simulink model "Model_6DOF_B3"  (R2020b)
settings: Solver=FixedStepAuto  StartTime=0.0  StopTime=120  FixedStep=0.05  RelTol=1e-3
values from neighbouring files (symbols this model uses):
  Ba_0 = [0 0 0 0 0 0]    [ctrl_mode_param.m]
  Bb = 4418825.3321    [load_data.m]
  Bv_0 = [tgt_speed 0 0 0 0 0]    [ctrl_mode_param.m]
  Bx_0 = [0 0 tgt_depth 0 0 0]    [ctrl_mode_param.m]
  Ixx = 5.23e7    (= 52300000)    [load_data.m]
  Ixy = 0    [load_data.m]
  Ixz = 0    [load_data.m]
  Iyy = 1.375e9    (= 1375000000)    [load_data.m]
  Iyz = 0    [load_data.m]
  Izz = 1.367e9    (= 1367000000)    [load_data.m]
  Mb = 4418825.3321    [load_data.m]
  Xb = 0    [load_data.m]
  Xg = 0    [load_data.m]
  Yb = 0    [load_data.m]
  Yg = 0    [load_data.m]
  Zb = 0.4406    [load_data.m]
  Zg = 0    [load_data.m]
undefined symbols (not defined in the file or in its folder): dA_BP1, dA_BP2, dA_Hull, dA_PH, dA_Sail, dA_SProot, dA_X1a, dA_X1b, dA_X2a, dA_X2b, dA_X3a, dA_X3b, dA_X4a, dA_X4b, its, n_BP1, n_BP2, n_Hull, n_PH, n_Sail, n_SProot, n_X1a, n_X1b, n_X2a, n_X2b, n_X3a, n_X3b, n_X4a, n_X4b, nt_BP1, nt_BP2, nt_Hull, nt_PH, nt_Sail, nt_SProot, nt_X1a, nt_X1b, nt_X2a, nt_X2b, nt_X3a, nt_X3b, nt_X4a, nt_X4b, Usp, vt1_BP1, vt1_BP2, vt1_Hull, vt1_PH, vt1_Sail, vt1_SProot, vt1_X1a, vt1_X1b, vt1_X2a, vt1_X2b, vt1_X3a, vt1_X3b, vt1_X4a, vt1_X4b, vt2_BP1, vt2_BP2 ... (+27)
libraries: simulink x5
(part 7 of 15)

== system Model_6DOF_B3/HDM 6DOF V1/X 6d org/Subsystem1 ==
  UeX : Inport
  dXeff : Inport  Port=2
  z : Inport  Port=3
  Demux : Demux  Outputs=5
  Demux1 : Demux  Outputs=5
  Mux : Mux  Inputs=5
  Xud4 : Lookup_n-D  NumberOfTableDimensions=3  BreakpointsForDimension1=[-30 -20 -10 0 10 20 30]  BreakpointsForDimension2=|  BreakpointsForDimension3=|  Table=|  InternalRulePriority=Speed  RndMeth=Simplest  InputSameDT=on
      BreakpointsForDimension2=|
      | [1.5433332
      | 3.0866664
      | 
      | 5.144444]
      BreakpointsForDimension3=|
      | [-36.3724
      | -18.3724
      | -15.3724
      | -13.8724]
      Table=|
      | reshape([1.9515E-04
      | 1.0370E-04
      | 3.9468E-05
      | 1.2612E-05
      | 3.9477E-05
      | 9.2497E-05
      | 1.9504E-04
      | 2.0037E-04
      | 9.3994E-05
      | 3.9650E-05
      | 1.2608E-05
      | 3.9217E-05
      | 9.5451E-05
      | 1.8893E-04
      | 2.0342E-04
      | 9.8349E-05
      | 3.9739E-05
      | 1.2608E-05
      | 3.9126E-05
      | 9.3002E-05
      | 1.9310E-04
      | 2.0342E-04
      | 9.7784E-05
      | 3.9737E-05
      | 1.2594E-05
      | 3.8955E-05
      | 9.3472E-05
      | 1.8818E-04
      | 1.9912E-04
      | 9.6216E-05
      | 3.8834E-05
      | 1.1823E-05
      | 3.8745E-05
      | 9.5316E-05
      | 1.9299E-04
      | 2.0055E-04
      | 9.7244E-05
      | 3.9050E-05
      | 1.1812E-05
      | 3.8434E-05
      | 9.0497E-05
      | 1.8966E-04
      | 2.6693E-04
      | 1.4022E-04
      | 3.8561E-05
      | 1.1822E-05
      | 3.3455E-05
      | 1.0520E-04
      | 2.4359E-04
      | 2.0044E-04
      | 1.0295E-04
      | 3.9158E-05
      | 1.1774E-05
      | 3.8178E-05
      | 9.0714E-05
      | 1.8818E-04
      | 1.9655E-04
      | 9.5339E-05
      | 3.8472E-05
      | 1.1287E-05
      | 3.8241E-05
      | 9.3683E-05
      | 1.8812E-04
      | 1.9890E-04
      | 9.7584E-05
      | 3.8662E-05
      | 1.1263E-05
      | 3.7865E-05
      | 8.8045E-05
      | 1.8986E-04
      | 2.6693E-04
      | 1.4022E-04
      | 3.8561E-05
      | 1.1263E-05
      | 3.3455E-05
      | 1.0520E-04
      | 2.4359E-04
      | 2.0199E-04
      | 9.6354E-05
      | 3.8835E-05
      | 1.1203E-05
      | 3.7555E-05
      | 8.7551E-05
      | 1.8761E-04],[7,3,4])
      settings: InputPortMap=u0,u1,u2
  XudX1 : Lookup_n-D  NumberOfTableDimensions=3  BreakpointsForDimension1=[-30 -20 -10 0 10 20 30]  BreakpointsForDimension2=|  BreakpointsForDimension3=|  Table=|  InternalRulePriority=Speed  RndMeth=Simplest  InputSameDT=on
      BreakpointsForDimension2=|
      | [1.5433332
      | 3.0866664
      | 
      | 5.144444]
      BreakpointsForDimension3=|
      | [-36.3724
      | -18.3724
      | -15.3724
      | -13.8724]
      Table=|
      | reshape([1.9726E-04
      | 9.2807E-05
      | 3.9153E-05
      | 1.2612E-05
      | 3.9108E-05
      | 9.6157E-05
      | 1.9721E-04
      | 1.9513E-04
      | 9.5505E-05
      | 3.8964E-05
      | 1.2607E-05
      | 3.9329E-05
      | 9.6357E-05
      | 1.9540E-04
      | 1.9473E-04
      | 1.0389E-04
      | 3.8933E-05
      | 1.2607E-05
      | 3.9448E-05
      | 9.9420E-05
      | 2.0231E-04
      | 1.9473E-04
      | 1.0019E-04
      | 3.8828E-05
      | 1.2592E-05
      | 3.9441E-05
      | 9.3211E-05
      | 2.0035E-04
      | 1.9312E-04
      | 9.4955E-05
      | 3.8460E-05
      | 1.1826E-05
      | 3.8411E-05
      | 9.3406E-05
      | 1.9672E-04
      | 1.9062E-04
      | 9.2834E-05
      | 3.8250E-05
      | 1.1814E-05
      | 3.8668E-05
      | 9.2911E-05
      | 1.9753E-04
      | 2.4353E-04
      | 1.0500E-04
      | 3.3326E-05
      | 1.1821E-05
      | 3.8282E-05
      | 1.3081E-04
      | 2.5995E-04
      | 1.8933E-04
      | 9.3556E-05
      | 3.8050E-05
      | 1.1773E-05
      | 3.8871E-05
      | 9.3887E-05
      | 2.0035E-04
      | 1.8690E-04
      | 9.6416E-05
      | 3.7999E-05
      | 1.1295E-05
      | 3.8027E-05
      | 9.1995E-05
      | 1.9449E-04
      | 1.9009E-04
      | 9.2479E-05
      | 3.7675E-05
      | 1.1269E-05
      | 3.8335E-05
      | 8.9889E-05
      | 1.9665E-04
      | 2.4353E-04
      | 1.0500E-04
      | 3.3326E-05
      | 1.1269E-05
      | 3.8282E-05
      | 1.3081E-04
      | 2.5995E-04
      | 1.8646E-04
      | 9.1163E-05
      | 3.7419E-05
      | 1.1206E-05
      | 3.8643E-05
      | 9.8736E-05
      | 2.0514E-04],[7,3,4])
      settings: InputPortMap=u0,u1,u2
  XudX1B : Lookup_n-D  NumberOfTableDimensions=3  BreakpointsForDimension1=[-30 -20 -10 0 10 20 30]  BreakpointsForDimension2=|  BreakpointsForDimension3=|  Table=|  InternalRulePriority=Speed  RndMeth=Simplest  InputSameDT=on
      BreakpointsForDimension2=|
      | [1.5433332
      | 3.0866664
      | 
      | 5.144444]
      BreakpointsForDimension3=|
      | [-36.3724
      | -18.3724
      | -15.3724
      | -13.8724]
      Table=|
      | reshape([3.9535E-04
      | 2.6403E-04
      | 1.4465E-04
      | 6.6976E-05
      | 1.2333E-04
      | 2.8515E-04
      | 3.5499E-04
      | 3.8973E-04
      | 2.6514E-04
      | 1.4731E-04
      | 6.8622E-05
      | 1.2628E-04
      | 2.9201E-04
      | 3.6632E-04
      | 4.0285E-04
      | 2.7250E-04
      | 1.4933E-04
      | 6.8622E-05
      | 1.2952E-04
      | 2.9373E-04
      | 3.6588E-04
      | 4.0285E-04
      | 2.8332E-04
      | 1.5162E-04
      | 7.2213E-05
      | 1.3467E-04
      | 3.0293E-04
      | 3.6349E-04
      | 3.8950E-04
      | 2.6292E-04
      | 1.4475E-04
      | 6.6785E-05
      | 1.2369E-04
      | 2.7281E-04
      | 3.4895E-04
      | 3.9519E-04
      | 2.6529E-04
      | 1.4760E-04
      | 6.8542E-05
      | 1.2717E-04
      | 2.7841E-04
      | 3.6301E-04
      | 5.6904E-04
      | 3.2107E-04
      | 1.3512E-04
      | 7.0542E-05
      | 1.0919E-04
      | 4.1259E-04
      | 6.2735E-04
      | 3.6838E-04
      | 3.0195E-04
      | 1.5438E-04
      | 7.4592E-05
      | 1.4048E-04
      | 3.1396E-04
      | 3.6349E-04
      | 4.1126E-04
      | 2.6224E-04
      | 1.4422E-04
      | 6.5961E-05
      | 1.2321E-04
      | 2.7802E-04
      | 3.5744E-04
      | 4.0057E-04
      | 2.6952E-04
      | 1.4782E-04
      | 6.8341E-05
      | 1.2789E-04
      | 2.8978E-04
      | 3.5944E-04
      | 5.6904E-04
      | 3.2107E-04
      | 1.3512E-04
      | 6.8341E-05
      | 1.0919E-04
      | 4.1259E-04
      | 6.2735E-04
      | 4.8319E-04
      | 3.1751E-04
      | 1.5761E-04
      | 7.4804E-05
      | 1.3557E-04
      | 3.2741E-04
      | 4.7146E-04],[7,3,4])
      settings: InputPortMap=u0,u1,u2
  XudX2 : Lookup_n-D  NumberOfTableDimensions=3  BreakpointsForDimension1=[-30 -20 -10 0 10 20 30]  BreakpointsForDimension2=|  BreakpointsForDimension3=|  Table=|  InternalRulePriority=Speed  RndMeth=Simplest  InputSameDT=on
      BreakpointsForDimension2=|
      | [1.5433332
      | 3.0866664
      | 
      | 5.144444]
      BreakpointsForDimension3=|
      | [-36.3724
      | -18.3724
      | -15.3724
      | -13.8724]
      Table=|
      | reshape([1.9988E-04
      | 9.2815E-05
      | 3.8984E-05
      | 1.2936E-05
      | 3.7333E-05
      | 1.0938E-04
      | 2.1913E-04
      | 2.0000E-04
      | 9.3101E-05
      | 3.8429E-05
      | 1.2739E-05
      | 3.7583E-05
      | 1.1064E-04
      | 2.1950E-04
      | 2.0083E-04
      | 9.4269E-05
      | 3.8054E-05
      | 1.2739E-05
      | 3.7662E-05
      | 1.0858E-04
      | 2.2083E-04
      | 2.0083E-04
      | 9.5605E-05
      | 3.7864E-05
      | 1.2538E-05
      | 3.7776E-05
      | 1.1595E-04
      | 2.1404E-04
      | 1.9933E-04
      | 9.2999E-05
      | 3.8198E-05
      | 1.2159E-05
      | 3.6475E-05
      | 1.0280E-04
      | 2.1737E-04
      | 2.0006E-04
      | 9.3307E-05
      | 3.7549E-05
      | 1.1957E-05
      | 3.6899E-05
      | 1.1530E-04
      | 2.2066E-04
      | 2.4216E-04
      | 1.0448E-04
      | 2.9342E-05
      | 1.1821E-05
      | 3.5012E-05
      | 1.3098E-04
      | 2.3359E-04
      | 1.9082E-04
      | 9.0828E-05
      | 3.6826E-05
      | 1.1709E-05
      | 3.7301E-05
      | 1.0927E-04
      | 2.1404E-04
      | 1.6701E-04
      | 9.2083E-05
      | 3.7750E-05
      | 1.1627E-05
      | 3.5975E-05
      | 9.9381E-05
      | 2.1803E-04
      | 1.9264E-04
      | 9.0003E-05
      | 3.6917E-05
      | 1.1397E-05
      | 3.6539E-05
      | 1.0523E-04
      | 2.1540E-04
      | 2.4216E-04
      | 1.0448E-04
      | 2.9342E-05
      | 1.1397E-05
      | 3.5012E-05
      | 1.3098E-04
      | 2.3359E-04
      | 1.8911E-04
      | 9.0019E-05
      | 3.6083E-05
      | 1.1213E-05
      | 3.7708E-05
      | 1.0882E-04
      | 1.6878E-04],[7,3,4])
      settings: InputPortMap=u0,u1,u2
  XudX3 : Lookup_n-D  NumberOfTableDimensions=3  BreakpointsForDimension1=[-30 -20 -10 0 10 20 30]  BreakpointsForDimension2=|  BreakpointsForDimension3=|  Table=|  InternalRulePriority=Speed  RndMeth=Simplest  InputSameDT=on
      BreakpointsForDimension2=|
      | [1.5433332
      | 3.0866664
      | 
      | 5.144444]
      BreakpointsForDimension3=|
      | [-36.3724
      | -18.3724
      | -15.3724
      | -13.8724]
      Table=|
      | reshape([2.1838E-04
      | 9.8768E-05
      | 3.9298E-05
      | 1.2921E-05
      | 4.0048E-05
      | 1.0549E-04
      | 1.8864E-04
      | 2.2881E-04
      | 1.0336E-04
      | 3.9060E-05
      | 1.2736E-05
      | 3.9535E-05
      | 1.0325E-04
      | 1.9538E-04
      | 2.1692E-04
      | 1.0227E-04
      | 3.8885E-05
      | 1.2736E-05
      | 3.9285E-05
      | 9.9666E-05
      | 1.9406E-04
      | 2.1692E-04
      | 1.0151E-04
      | 3.8619E-05
      | 1.2552E-05
      | 3.9212E-05
      | 1.0291E-04
      | 2.0160E-04
      | 2.1667E-04
      | 1.0323E-04
      | 3.9049E-05
      | 1.2140E-05
      | 3.9810E-05
      | 1.0079E-04
      | 1.9039E-04
      | 2.2496E-04
      | 9.9708E-05
      | 3.8786E-05
      | 1.1948E-05
      | 3.9280E-05
      | 1.0040E-04
      | 1.8622E-04
      | 2.7315E-04
      | 1.3714E-04
      | 3.4983E-05
      | 1.1821E-05
      | 3.1018E-05
      | 1.0427E-04
      | 1.9674E-04
      | 2.2211E-04
      | 1.0444E-04
      | 3.8528E-05
      | 1.1713E-05
      | 3.8636E-05
      | 9.5401E-05
      | 2.0160E-04
      | 2.0348E-04
      | 1.0451E-04
      | 3.8863E-05
      | 1.1608E-05
      | 3.9501E-05
      | 1.0479E-04
      | 1.8840E-04
      | 2.0541E-04
      | 9.7216E-05
      | 3.8561E-05
      | 1.1388E-05
      | 3.8824E-05
      | 9.5169E-05
      | 1.8576E-04
      | 2.7315E-04
      | 1.3714E-04
      | 3.4983E-05
      | 1.1388E-05
      | 3.1018E-05
      | 1.0427E-04
      | 1.9674E-04
      | 2.1961E-04
      | 1.1536E-04
      | 3.8716E-05
      | 1.1221E-05
      | 3.7813E-05
      | 9.5976E-05
      | 1.9612E-04],[7,3,4])
      settings: InputPortMap=u0,u1,u2
  XdXi : Outport
  wires:
  Mux/1 -> XdXi/1
  XudX1/1 -> Mux/1
  XudX2/1 -> Mux/2
  Xud4/1 -> Mux/4
  dXeff/1 -> Demux1/1
  UeX/1 -> Demux/1
  XudX3/1 -> Mux/3
  XudX1B/1 -> Mux/5
  Demux/1 -> XudX1/2
  Demux/2 -> XudX2/2
  Demux/3 -> XudX3/2
  Demux/4 -> Xud4/2
  Demux/5 -> XudX1B/2
  z/1 -> XudX1/3, XudX2/3, XudX3/3, XudX1B/3, Xud4/3
  Demux1/1 -> XudX1/1
  Demux1/2 -> XudX2/1
  Demux1/3 -> XudX3/1
  Demux1/5 -> XudX1B/1
  Demux1/4 -> Xud4/1

== system Model_6DOF_B3/HDM 6DOF V1/Y/YdXi ==
  dX : Inport
  z : Inport  Port=2
  Mux : Mux
  Selector1 : Selector  InputPortWidth=5  IndexOptions=Index vector (dialog)  Indices=2  OutputSizes=1
  Selector2 : Selector  InputPortWidth=5  IndexOptions=Index vector (dialog)  Indices=3  OutputSizes=1
  Selector3 : Selector  InputPortWidth=5  IndexOptions=Index vector (dialog)  Indices=4  OutputSizes=1
  Selector7 : Selector  InputPortWidth=5  IndexOptions=Index vector (dialog)  Indices=1  OutputSizes=1
  YdX1 : Lookup_n-D  BreakpointsForDimension1=[-10 0 10]  BreakpointsForDimension2=|  BreakpointsForDimension3=[-5.14444 -3.08666664 -1.54332]  Table=|  InternalRulePriority=Speed  RndMeth=Simplest  InputSameDT=on
      BreakpointsForDimension2=|
      | [-36.4062987
      | -18.4062987
      | -15.4062987
      | -13.9062987]
      Table=|
      | reshape([-1.8282E-04
      | -6.0037E-06
      | 1.6496E-04
      | -1.7978E-04
      | -2.4314E-06
      | 1.6969E-04
      | -1.4480E-04
      | -2.4314E-06
      | 2.0267E-04
      | -1.7641E-04
      | 1.4850E-06
      | 1.7514E-04],[3,4])
      settings: InputPortMap=u0,u1
  YdX2 : Lookup_n-D  BreakpointsForDimension1=[-10 0 10]  BreakpointsForDimension2=|  BreakpointsForDimension3=[-5.14444 -3.08666664 -1.54332]  Table=|  InternalRulePriority=Speed  RndMeth=Simplest  InputSameDT=on
      BreakpointsForDimension2=|
      | [-36.4062987
      | -18.4062987
      | -15.4062987
      | -13.9062987]
      Table=|
      | reshape([1.4857E-04
      | -6.6611E-06
      | -1.5932E-04
      | 1.4200E-04
      | -1.2968E-05
      | -1.6860E-04
      | 9.4982E-05
      | -1.2968E-05
      | -2.1344E-04
      | 1.3366E-04
      | -2.3176E-05
      | -1.8599E-04],[3,4])
      settings: InputPortMap=u0,u1
  YdX3 : Lookup_n-D  BreakpointsForDimension1=[-10 0 10]  BreakpointsForDimension2=|  BreakpointsForDimension3=[-5.14444 -3.08666664 -1.54332]  Table=|  InternalRulePriority=Speed  RndMeth=Simplest  InputSameDT=on
      BreakpointsForDimension2=|
      | [-36.4062987
      | -18.4062987
      | -15.4062987
      | -13.9062987]
      Table=|
      | reshape([2.0207E-04
      | 6.9701E-06
      | -1.9141E-04
      | 2.0588E-04
      | 1.3213E-05
      | -1.8007E-04
      | 2.2753E-04
      | 1.3213E-05
      | -1.0937E-04
      | 2.1222E-04
      | 2.3270E-05
      | -1.6161E-04],[3,4])
      settings: InputPortMap=u0,u1
  YdX4 : Lookup_n-D  BreakpointsForDimension1=[-10 0 10]  BreakpointsForDimension2=|  BreakpointsForDimension3=[-5.14444 -3.08666664 -1.54332]  Table=|  InternalRulePriority=Speed  RndMeth=Simplest  InputSameDT=on
      BreakpointsForDimension2=|
      | [-36.4062987
      | -18.4062987
      | -15.4062987
      | -13.9062987]
      Table=|
      | reshape([-1.7022E-04
      | 5.9932E-06
      | 1.8722E-04
      | -1.7390E-04
      | 2.3770E-06
      | 1.8293E-04
      | -2.0489E-04
      | 2.3770E-06
      | 1.4658E-04
      | -1.7771E-04
      | -1.6689E-06
      | 1.7805E-04],[3,4])
      settings: InputPortMap=u0,u1
  YdX : Outport
  wires:
  Mux/1 -> YdX/1
  z/1 -> YdX4/2, YdX3/2, YdX2/2, YdX1/2
  YdX1/1 -> Mux/1
  YdX2/1 -> Mux/2
  YdX3/1 -> Mux/3
  YdX4/1 -> Mux/4
  Selector7/1 -> YdX1/1
  dX/1 -> Selector2/1, Selector3/1, Selector1/1, Selector7/1
  Selector3/1 -> YdX4/1
  Selector2/1 -> YdX3/1
  Selector1/1 -> YdX2/1

== system Model_6DOF_B3/HDM 6DOF V1/Z/ZdXi ==
  dX : Inport
  z : Inport  Port=2
  Demux6 : Demux  Outputs=5
  Mux : Mux  Inputs=5
  ZudX1 q+10 : Lookup_n-D  BreakpointsForDimension1=[-30 -20 -10 0 10 20 30]  BreakpointsForDimension2=[-35.0624 -15.3724 -13.8724]  BreakpointsForDimension3=[-35.0624 -15.3724 -13.8724]  Table=|  InternalRulePriority=Speed  RndMeth=Simplest  InputSameDT=on
      | reshape([-0.003226964
      | -0.002116041
      | -0.001005119
      | 0.000105803
      | 0.001216725
      | 0.002327647
      | 0.003438569
      | -0.003036597
      | -0.001876165
      | -0.000715732
      | 0.0004447
      | 0.001605132
      | 0.002765565
      | 0.003925997
      | -0.003676642
      | -0.002490275
      | -0.001303908
      | -0.000117541
      | 0.001068826
      | 0.002255193
      | 0.00344156],[7,3])
      settings: InputPortMap=u0,u1
  ZudX1 q+6 : Lookup_n-D  BreakpointsForDimension1=[-30 -20 -10 0 10 20 30]  BreakpointsForDimension2=[-35.0624 -15.3724 -13.8724]  BreakpointsForDimension3=[-5.14444 -3.08666664 -1.54332]  Table=|  InternalRulePriority=Speed  RndMeth=Simplest  InputSameDT=on
      | reshape([-0.001383757
      | -0.000911
      | -0.000438243
      | 3.45135E-05
      | 0.00050727
      | 0.000980027
      | 0.001452784
      | -0.001383757
      | -0.000911
      | -0.000438243
      | 3.45135E-05
      | 0.00050727
      | 0.000980027
      | 0.001452784
      | -0.001353354
      | -0.000887631
      | -0.000421908
      | 4.38143E-05
      | 0.000509537
      | 0.00097526
      | 0.001440982],[7,3])
      settings: InputPortMap=u0,u1
  ZudX1 q+7 : Lookup_n-D  BreakpointsForDimension1=[-30 -20 -10 0 10 20 30]  BreakpointsForDimension2=[-35.0624 -15.3724 -13.8724]  BreakpointsForDimension3=[-5.14444 -3.08666664 -1.54332]  Table=|  InternalRulePriority=Speed  RndMeth=Simplest  InputSameDT=on
      | reshape([-0.001358511
      | -0.00091651
      | -0.000474508
      | -3.25062E-05
      | 0.000409495
      | 0.000851497
      | 0.001293499
      | -0.001303275
      | -0.00086798
      | -0.000432686
      | 2.60877E-06
      | 0.000437903
      | 0.000873198
      | 0.001308493
      | -0.001263287
      | -0.000836064
      | -0.00040884
      | 1.83841E-05
      | 0.000445608
      | 0.000872832
      | 0.001300056],[7,3])
      settings: InputPortMap=u0,u1
  ZudX1 q+8 : Lookup_n-D  BreakpointsForDimension1=[-30 -20 -10 0 10 20 30]  BreakpointsForDimension2=[-35.0624 -15.3724 -13.8724]  BreakpointsForDimension3=[-5.14444 -3.08666664 -1.54332]  Table=|  InternalRulePriority=Speed  RndMeth=Simplest  InputSameDT=on
      | reshape([0.001309084
      | 0.000864124
      | 0.000419163
      | -2.5798E-05
      | -0.000470759
      | -0.000915719
      | -0.00136068
      | 0.001321953
      | 0.000882434
      | 0.000442915
      | 3.39516E-06
      | -0.000436124
      | -0.000875644
      | -0.001315163
      | 0.001313186
      | 0.000881448
      | 0.000449709
      | 1.79712E-05
      | -0.000413767
      | -0.000845505
      | -0.001277243],[7,3])
      settings: InputPortMap=u0,u1
  ZudX1 q+9 : Lookup_n-D  BreakpointsForDimension1=[-30 -20 -10 0 10 20 30]  BreakpointsForDimension2=[-35.0624 -15.3724 -13.8724]  BreakpointsForDimension3=[-5.14444 -3.08666664 -1.54332]  Table=|  InternalRulePriority=Speed  RndMeth=Simplest  InputSameDT=on
      | reshape([0.001464336
      | 0.000977857
      | 0.000491377
      | 4.89775E-06
      | -0.000481582
      | -0.000968061
      | -0.00145454
      | 0.001455937
      | 0.00098192
      | 0.000507903
      | 3.38863E-05
      | -0.00044013
      | -0.000914147
      | -0.001388164
      | 0.001460604
      | 0.00098818
      | 0.000515756
      | 4.33325E-05
      | -0.000429091
      | -0.000901515
      | -0.001373939],[7,3])
      settings: InputPortMap=u0,u1
  ZdX : Outport
  wires:
  ZudX1 q+9/1 -> Mux/4
  ZudX1 q+8/1 -> Mux/3
  ZudX1 q+7/1 -> Mux/2
  ZudX1 q+6/1 -> Mux/1
  ZudX1 q+10/1 -> Mux/5
  z/1 -> ZudX1 q+9/2, ZudX1 q+10/2, ZudX1 q+8/2, ZudX1 q+7/2, ZudX1 q+6/2
  Demux6/5 -> ZudX1 q+10/1
  Mux/1 -> ZdX/1
  Demux6/1 -> ZudX1 q+6/1
  Demux6/2 -> ZudX1 q+7/1
  Demux6/4 -> ZudX1 q+9/1
  dX/1 -> Demux6/1
  Demux6/3 -> ZudX1 q+8/1

== system Model_6DOF_B3/HDM 6DOF V1/Z 6d org/ZdXi ==
  dX : Inport
  z : Inport  Port=2
  Demux6 : Demux  Outputs=5
  Mux : Mux  Inputs=5
  ZudX1 q+10 : Lookup_n-D  BreakpointsForDimension1=[-30 -20 -10 0 10 20 30]  BreakpointsForDimension2=[-35.0624 -15.3724 -13.8724]  BreakpointsForDimension3=[-35.0624 -15.3724 -13.8724]  Table=|  InternalRulePriority=Speed  RndMeth=Simplest  InputSameDT=on
      | reshape([-0.003226964
      | -0.002116041
      | -0.001005119
      | 0.000105803
      | 0.001216725
      | 0.002327647
      | 0.003438569
      | -0.003036597
      | -0.001876165
      | -0.000715732
      | 0.0004447
      | 0.001605132
      | 0.002765565
      | 0.003925997
      | -0.003676642
      | -0.002490275
      | -0.001303908
      | -0.000117541
      | 0.001068826
      | 0.002255193
      | 0.00344156],[7,3])
      settings: InputPortMap=u0,u1
  ZudX1 q+6 : Lookup_n-D  BreakpointsForDimension1=[-30 -20 -10 0 10 20 30]  BreakpointsForDimension2=[-35.0624 -15.3724 -13.8724]  BreakpointsForDimension3=[-5.14444 -3.08666664 -1.54332]  Table=|  InternalRulePriority=Speed  RndMeth=Simplest  InputSameDT=on
      | reshape([-0.001383757
      | -0.000911
      | -0.000438243
      | 3.45135E-05
      | 0.00050727
      | 0.000980027
      | 0.001452784
      | -0.001383757
      | -0.000911
      | -0.000438243
      | 3.45135E-05
      | 0.00050727
      | 0.000980027
      | 0.001452784
      | -0.001353354
      | -0.000887631
      | -0.000421908
      | 4.38143E-05
      | 0.000509537
      | 0.00097526
      | 0.001440982],[7,3])
      settings: InputPortMap=u0,u1
  ZudX1 q+7 : Lookup_n-D  BreakpointsForDimension1=[-30 -20 -10 0 10 20 30]  BreakpointsForDimension2=[-35.0624 -15.3724 -13.8724]  BreakpointsForDimension3=[-5.14444 -3.08666664 -1.54332]  Table=|  InternalRulePriority=Speed  RndMeth=Simplest  InputSameDT=on
      | reshape([-0.001358511
      | -0.00091651
      | -0.000474508
      | -3.25062E-05
      | 0.000409495
      | 0.000851497
      | 0.001293499
      | -0.001303275
      | -0.00086798
      | -0.000432686
      | 2.60877E-06
      | 0.000437903
      | 0.000873198
      | 0.001308493
      | -0.001263287
      | -0.000836064
      | -0.00040884
      | 1.83841E-05
      | 0.000445608
      | 0.000872832
      | 0.001300056],[7,3])
      settings: InputPortMap=u0,u1
  ZudX1 q+8 : Lookup_n-D  BreakpointsForDimension1=[-30 -20 -10 0 10 20 30]  BreakpointsForDimension2=[-35.0624 -15.3724 -13.8724]  BreakpointsForDimension3=[-5.14444 -3.08666664 -1.54332]  Table=|  InternalRulePriority=Speed  RndMeth=Simplest  InputSameDT=on
      | reshape([0.001309084
      | 0.000864124
      | 0.000419163
      | -2.5798E-05
      | -0.000470759
      | -0.000915719
      | -0.00136068
      | 0.001321953
      | 0.000882434
      | 0.000442915
      | 3.39516E-06
      | -0.000436124
      | -0.000875644
      | -0.001315163
      | 0.001313186
      | 0.000881448
      | 0.000449709
      | 1.79712E-05
      | -0.000413767
      | -0.000845505
      | -0.001277243],[7,3])
      settings: InputPortMap=u0,u1
  ZudX1 q+9 : Lookup_n-D  BreakpointsForDimension1=[-30 -20 -10 0 10 20 30]  BreakpointsForDimension2=[-35.0624 -15.3724 -13.8724]  BreakpointsForDimension3=[-5.14444 -3.08666664 -1.54332]  Table=|  InternalRulePriority=Speed  RndMeth=Simplest  InputSameDT=on
      | reshape([0.001464336
      | 0.000977857
      | 0.000491377
      | 4.89775E-06
      | -0.000481582
      | -0.000968061
      | -0.00145454
      | 0.001455937
      | 0.00098192
      | 0.000507903
      | 3.38863E-05
      | -0.00044013
      | -0.000914147
      | -0.001388164
      | 0.001460604
      | 0.00098818
      | 0.000515756
      | 4.33325E-05
      | -0.000429091
      | -0.000901515
      | -0.001373939],[7,3])
      settings: InputPortMap=u0,u1
  ZdX : Outport
  wires:
  Demux6/3 -> ZudX1 q+8/1
  dX/1 -> Demux6/1
  Demux6/4 -> ZudX1 q+9/1
  Demux6/2 -> ZudX1 q+7/1
  Demux6/1 -> ZudX1 q+6/1
  Demux6/5 -> ZudX1 q+10/1
  z/1 -> ZudX1 q+10/2, ZudX1 q+9/2, ZudX1 q+8/2, ZudX1 q+7/2, ZudX1 q+6/2
  ZudX1 q+10/1 -> Mux/5
  ZudX1 q+6/1 -> Mux/1
  ZudX1 q+7/1 -> Mux/2
  ZudX1 q+8/1 -> Mux/3
  ZudX1 q+9/1 -> Mux/4
  Mux/1 -> ZdX/1

== system Model_6DOF_B3/HDM B1/K/KdXi ==
  dX : Inport
  UeX : Inport  Port=2
  z : Inport  Port=3
  KdX1 : Lookup_n-D  NumberOfTableDimensions=3  BreakpointsForDimension1=[-10 0 10]  BreakpointsForDimension2=|  BreakpointsForDimension3=[-5.14444 -3.08666664 -1.54332]  Table=|  InternalRulePriority=Speed  RndMeth=Simplest  InputSameDT=on
      BreakpointsForDimension2=|
      | [-36.4062987
      | -18.4062987
      | -15.4062987
      | -13.9062987]
      Table=|
      | reshape([-3.9047E-05
      | 4.5684E-07
      | 3.9769E-05
      | -3.8309E-05
      | 1.2643E-06
      | 4.0809E-05
      | -3.0256E-05
      | 1.2643E-06
      | 4.8387E-05
      | -3.7558E-05
      | 2.1545E-06
      | 4.2083E-05
      | -3.9057E-05
      | 3.6064E-07
      | 3.9562E-05
      | -3.8473E-05
      | 1.0476E-06
      | 4.0437E-05
      | -3.0256E-05
      | 1.4418E-06
      | 4.8387E-05
      | -3.7906E-05
      | 1.7415E-06
      | 4.1434E-05
      | -3.8945E-05
      | 2.8249E-07
      | 3.9429E-05
      | -3.8396E-05
      | 9.1134E-07
      | 4.0237E-05
      | -3.8190E-05
      | 9.1134E-07
      | 4.0733E-05
      | -3.7932E-05
      | 1.5343E-06
      | 4.1020E-05
      | ],[3,4,3])
      settings: InputPortMap=u0,u1,u2
  KdX2 : Lookup_n-D  NumberOfTableDimensions=3  BreakpointsForDimension1=[-10 0 10]  BreakpointsForDimension2=|  BreakpointsForDimension3=[-5.14444 -3.08666664 -1.54332]  Table=|  InternalRulePriority=Speed  RndMeth=Simplest  InputSameDT=on
      BreakpointsForDimension2=|
      | [-36.4062987
      | -18.4062987
      | -15.4062987
      | -13.9062987]
      Table=|
      | reshape([-3.5775E-05
      | -2.4080E-07
      | 3.3150E-05
      | -3.4263E-05
      | 1.2268E-06
      | 3.5342E-05
      | -2.3577E-05
      | 1.2268E-06
      | 4.6338E-05
      | -3.2368E-05
      | 3.5682E-06
      | 3.9469E-05
      | -3.5785E-05
      | -3.3131E-07
      | 3.3067E-05
      | -3.4544E-05
      | 8.9010E-07
      | 3.4889E-05
      | -2.3577E-05
      | 1.7076E-06
      | 4.6338E-05
      | -3.3141E-05
      | 2.4187E-06
      | 3.7389E-05
      | -3.5809E-05
      | -5.7189E-07
      | 3.3046E-05
      | -3.4706E-05
      | 4.2723E-07
      | 3.4588E-05
      | -3.4017E-05
      | 4.2723E-07
      | 3.5657E-05
      | -3.3562E-05
      | 1.6134E-06
      | 3.6605E-05
      | ],[3,4,3])
      settings: InputPortMap=u0,u1,u2
  KdX3 : Lookup_n-D  NumberOfTableDimensions=3  BreakpointsForDimension1=[-10 0 10]  BreakpointsForDimension2=|  BreakpointsForDimension3=[-5.14444 -3.08666664 -1.54332]  Table=|  InternalRulePriority=Speed  RndMeth=Simplest  InputSameDT=on
      BreakpointsForDimension2=|
      | [-36.4062987
      | -18.4062987
      | -15.4062987
      | -13.9062987]
      Table=|
      | reshape([-4.3139E-05
      | 1.7292E-07
      | 4.5001E-05
      | -4.4081E-05
      | -1.2796E-06
      | 4.2448E-05
      | -4.9749E-05
      | -1.2796E-06
      | 2.6691E-05
      | -4.5613E-05
      | -3.5861E-06
      | 3.8362E-05
      | -4.2707E-05
      | 2.7384E-07
      | 4.4575E-05
      | -4.3360E-05
      | -9.3523E-07
      | 4.2465E-05
      | -4.9749E-05
      | -1.7362E-06
      | 2.6691E-05
      | -4.4279E-05
      | -2.4363E-06
      | 3.9821E-05
      | -4.1687E-05
      | 5.3371E-07
      | 4.3082E-05
      | -4.2289E-05
      | -4.5361E-07
      | 4.1207E-05
      | -4.2616E-05
      | -4.5361E-07
      | 4.0204E-05
      | -4.2521E-05
      | -1.6159E-06
      | 3.9463E-05
      | ],[3,4,3])
      settings: InputPortMap=u0,u1,u2
  KdX4 : Lookup_n-D  NumberOfTableDimensions=3  BreakpointsForDimension1=[-10 0 10]  BreakpointsForDimension2=|  BreakpointsForDimension3=[-5.14444 -3.08666664 -1.54332]  Table=|  InternalRulePriority=Speed  RndMeth=Simplest  InputSameDT=on
      BreakpointsForDimension2=|
      | [-36.4062987
      | -18.4062987
      | -15.4062987
      | -13.9062987]
      Table=|
      | reshape([-4.0969E-05
      | -4.5313E-07
      | 4.0019E-05
      | -4.1787E-05
      | -1.2714E-06
      | 3.9006E-05
      | -4.8908E-05
      | -1.2714E-06
      | 3.0663E-05
      | -4.2681E-05
      | -2.1920E-06
      | 3.7920E-05
      | -4.0777E-05
      | -3.6185E-07
      | 4.0047E-05
      | -4.1470E-05
      | -1.0577E-06
      | 3.9147E-05
      | -4.8908E-05
      | -1.4679E-06
      | 3.0663E-05
      | -4.2187E-05
      | -1.7779E-06
      | 3.8312E-05
      | -4.0496E-05
      | -2.8854E-07
      | 4.0049E-05
      | -4.1082E-05
      | -9.2714E-07
      | 3.9223E-05
      | -4.1472E-05
      | -9.2714E-07
      | 3.8784E-05
      | -4.1733E-05
      | -1.5768E-06
      | 3.8383E-05
      | ],[3,4,3])
      settings: InputPortMap=u0,u1,u2
  Mux : Mux
  Selector1 : Selector  InputPortWidth=5  IndexOptions=Index vector (dialog)  Indices=2  OutputSizes=1
  Selector2 : Selector  InputPortWidth=5  IndexOptions=Index vector (dialog)  Indices=3  OutputSizes=1
  Selector3 : Selector  InputPortWidth=5  IndexOptions=Index vector (dialog)  Indices=4  OutputSizes=1
  Selector4 : Selector  InputPortWidth=5  IndexOptions=Index vector (dialog)  Indices=1  OutputSizes=1
  Selector5 : Selector  InputPortWidth=5  IndexOptions=Index vector (dialog)  Indices=2  OutputSizes=1
  Selector6 : Selector  InputPortWidth=5  IndexOptions=Index vector (dialog)  Indices=3  OutputSizes=1
  Selector7 : Selector  InputPortWidth=5  IndexOptions=Index vector (dialog)  Indices=1  OutputSizes=1
  Selector8 : Selector  InputPortWidth=5  IndexOptions=Index vector (dialog)  Indices=4  OutputSizes=1
  KdXi : Outport
  wires:
  Selector5/1 -> KdX2/3
  Selector6/1 -> KdX3/3
  Selector8/1 -> KdX4/3
  Selector4/1 -> KdX1/3
  UeX/1 -> Selector4/1, Selector5/1, Selector8/1, Selector6/1
  Selector3/1 -> KdX4/1
  Selector2/1 -> KdX3/1
  Selector1/1 -> KdX2/1
  KdX4/1 -> Mux/4
  KdX3/1 -> Mux/3
  KdX2/1 -> Mux/2
  KdX1/1 -> Mux/1
  z/1 -> KdX1/2, KdX2/2, KdX3/2, KdX4/2
  Mux/1 -> KdXi/1
  Selector7/1 -> KdX1/1
  dX/1 -> Selector7/1, Selector2/1, Selector3/1, Selector1/1

== system Model_6DOF_B3/HDM B1/M/Mdxi ==
  dX : Inport
  z : Inport  Port=2
  Demux6 : Demux  Outputs=5
  Gain{,1..4} (5 alike) : Gain
  Mux : Mux  Inputs=5
  ZudX1 q+1 : Lookup_n-D  BreakpointsForDimension1=[-30 -20 -10 0 10 20 30]  BreakpointsForDimension2=[-35.0624 -15.3724 -13.8724]  BreakpointsForDimension3=[-5.14444 -3.08666664 -1.54332]  Table=|  InternalRulePriority=Speed  RndMeth=Simplest  InputSameDT=on
      | reshape([0.000594819
      | 0.000394915
      | 0.000195011
      | -4.89222E-06
      | -0.000204796
      | -0.0004047
      | -0.000604603
      | 0.000596203
      | 0.000392018
      | 0.000187833
      | -1.6352E-05
      | -0.000220537
      | -0.000424722
      | -0.000628907
      | 0.000582351
      | 0.000381446
      | 0.000180542
      | -2.03625E-05
      | -0.000221267
      | -0.000422171
      | -0.000623076
      | ],[7,3])
      settings: InputPortMap=u0,u1
  ZudX1 q+2 : Lookup_n-D  BreakpointsForDimension1=[-30 -20 -10 0 10 20 30]  BreakpointsForDimension2=[-35.0624 -15.3724 -13.8724]  BreakpointsForDimension3=[-5.14444 -3.08666664 -1.54332]  Table=|  InternalRulePriority=Speed  RndMeth=Simplest  InputSameDT=on
      | reshape([0.000583784
      | 0.000394316
      | 0.000204847
      | 1.53782E-05
      | -0.000174091
      | -0.000363559
      | -0.000553028
      | 0.00056228
      | 0.000374724
      | 0.000187169
      | -3.86644E-07
      | -0.000187942
      | -0.000375498
      | -0.000563053
      | 0.000546298
      | 0.000362052
      | 0.000177806
      | -6.43933E-06
      | -0.000190685
      | -0.000374931
      | -0.000559176],[7,3])
      settings: InputPortMap=u0,u1
  ZudX1 q+3 : Lookup_n-D  BreakpointsForDimension1=[-30 -20 -10 0 10 20 30]  BreakpointsForDimension2=[-35.0624 -15.3724 -13.8724]  BreakpointsForDimension3=[-5.14444 -3.08666664 -1.54332]  Table=|  InternalRulePriority=Speed  RndMeth=Simplest  InputSameDT=on
      | reshape([-0.000586989
      | -0.000395541
      | -0.000204094
      | -1.26467E-05
      | 0.000178801
      | 0.000370248
      | 0.000561695
      | -0.000568868
      | -0.000379268
      | -0.000189669
      | -6.86388E-08
      | 0.000189531
      | 0.000379131
      | 0.000568731
      | -0.000565299
      | -0.000378949
      | -0.000192598
      | -6.24776E-06
      | 0.000180103
      | 0.000366453
      | 0.000552804],[7,3])
      settings: InputPortMap=u0,u1
  ZudX1 q+4 : Lookup_n-D  BreakpointsForDimension1=[-30 -20 -10 0 10 20 30]  BreakpointsForDimension2=[-35.0624 -15.3724 -13.8724]  BreakpointsForDimension3=[-5.14444 -3.08666664 -1.54332]  Table=|  InternalRulePriority=Speed  RndMeth=Simplest  InputSameDT=on
      | reshape([-0.000638396
      | -0.000426715
      | -0.000215035
      | -3.35454E-06
      | 0.000208326
      | 0.000420006
      | 0.000631687
      | -0.000598951
      | -0.000393944
      | -0.000188937
      | 1.60698E-05
      | 0.000221077
      | 0.000426084
      | 0.000631091
      | -0.000622514
      | -0.000421726
      | -0.000220939
      | -2.01522E-05
      | 0.000180635
      | 0.000381422
      | 0.000582209],[7,3])
      settings: InputPortMap=u0,u1
  ZudX1 q+5 : Lookup_n-D  BreakpointsForDimension1=[-30 -20 -10 0 10 20 30]  BreakpointsForDimension2=[-35.0624 -15.3724 -13.8724]  BreakpointsForDimension3=[-35.0624 -15.3724 -13.8724]  Table=|  InternalRulePriority=Speed  RndMeth=Simplest  InputSameDT=on
      | reshape([-0.000461714
      | -0.000296336
      | -0.000130959
      | 3.44194E-05
      | 0.000199797
      | 0.000365175
      | 0.000530553
      | -0.000503641
      | -0.000327652
      | -0.000151663
      | 2.43257E-05
      | 0.000200315
      | 0.000376303
      | 0.000552292
      | -0.000536558
      | -0.000356664
      | -0.00017677
      | 3.1235E-06
      | 0.000183017
      | 0.000362911
      | 0.000542805],[7,3])
      settings: InputPortMap=u0,u1
  MdX : Outport
  wires:
  Gain4/1 -> Mux/5
  Gain1/1 -> Mux/4
  Gain2/1 -> Mux/3
  Gain3/1 -> Mux/2
  Gain/1 -> Mux/1
  dX/1 -> Demux6/1
  Demux6/1 -> ZudX1 q+1/1
  Mux/1 -> MdX/1
  z/1 -> ZudX1 q+1/2, ZudX1 q+2/2, ZudX1 q+3/2, ZudX1 q+4/2, ZudX1 q+5/2
  ZudX1 q+5/1 -> Gain4/1
  ZudX1 q+1/1 -> Gain/1
  ZudX1 q+2/1 -> Gain3/1
  ZudX1 q+3/1 -> Gain2/1
  ZudX1 q+4/1 -> Gain1/1
  Demux6/2 -> ZudX1 q+2/1
  Demux6/3 -> ZudX1 q+3/1
  Demux6/4 -> ZudX1 q+4/1
  Demux6/5 -> ZudX1 q+5/1

== system Model_6DOF_B3/HDM B1/M 6d org/Mdxi ==
  dX : Inport
  z : Inport  Port=2
  Demux6 : Demux  Outputs=5
  Mux : Mux  Inputs=5
  ZudX1 q+1 : Lookup_n-D  BreakpointsForDimension1=[-30 -20 -10 0 10 20 30]  BreakpointsForDimension2=[-35.0624 -15.3724 -13.8724]  BreakpointsForDimension3=[-5.14444 -3.08666664 -1.54332]  Table=|  InternalRulePriority=Speed  RndMeth=Simplest  InputSameDT=on
      | reshape([0.000594819
      | 0.000394915
      | 0.000195011
      | -4.89222E-06
      | -0.000204796
      | -0.0004047
      | -0.000604603
      | 0.000596203
      | 0.000392018
      | 0.000187833
      | -1.6352E-05
      | -0.000220537
      | -0.000424722
      | -0.000628907
      | 0.000582351
      | 0.000381446
      | 0.000180542
      | -2.03625E-05
      | -0.000221267
      | -0.000422171
      | -0.000623076
      | ],[7,3])
      settings: InputPortMap=u0,u1
  ZudX1 q+2 : Lookup_n-D  BreakpointsForDimension1=[-30 -20 -10 0 10 20 30]  BreakpointsForDimension2=[-35.0624 -15.3724 -13.8724]  BreakpointsForDimension3=[-5.14444 -3.08666664 -1.54332]  Table=|  InternalRulePriority=Speed  RndMeth=Simplest  InputSameDT=on
      | reshape([0.000583784
      | 0.000394316
      | 0.000204847
      | 1.53782E-05
      | -0.000174091
      | -0.000363559
      | -0.000553028
      | 0.00056228
      | 0.000374724
      | 0.000187169
      | -3.86644E-07
      | -0.000187942
      | -0.000375498
      | -0.000563053
      | 0.000546298
      | 0.000362052
      | 0.000177806
      | -6.43933E-06
      | -0.000190685
      | -0.000374931
      | -0.000559176],[7,3])
      settings: InputPortMap=u0,u1
  ZudX1 q+3 : Lookup_n-D  BreakpointsForDimension1=[-30 -20 -10 0 10 20 30]  BreakpointsForDimension2=[-35.0624 -15.3724 -13.8724]  BreakpointsForDimension3=[-5.14444 -3.08666664 -1.54332]  Table=|  InternalRulePriority=Speed  RndMeth=Simplest  InputSameDT=on
      | reshape([-0.000586989
      | -0.000395541
      | -0.000204094
      | -1.26467E-05
      | 0.000178801
      | 0.000370248
      | 0.000561695
      | -0.000568868
      | -0.000379268
      | -0.000189669
      | -6.86388E-08
      | 0.000189531
      | 0.000379131
      | 0.000568731
      | -0.000565299
      | -0.000378949
      | -0.000192598
      | -6.24776E-06
      | 0.000180103
      | 0.000366453
      | 0.000552804],[7,3])
      settings: InputPortMap=u0,u1
  ZudX1 q+4 : Lookup_n-D  BreakpointsForDimension1=[-30 -20 -10 0 10 20 30]  BreakpointsForDimension2=[-35.0624 -15.3724 -13.8724]  BreakpointsForDimension3=[-5.14444 -3.08666664 -1.54332]  Table=|  InternalRulePriority=Speed  RndMeth=Simplest  InputSameDT=on
      | reshape([-0.000638396
      | -0.000426715
      | -0.000215035
      | -3.35454E-06
      | 0.000208326
      | 0.000420006
      | 0.000631687
      | -0.000598951
      | -0.000393944
      | -0.000188937
      | 1.60698E-05
      | 0.000221077
      | 0.000426084
      | 0.000631091
      | -0.000622514
      | -0.000421726
      | -0.000220939
      | -2.01522E-05
      | 0.000180635
      | 0.000381422
      | 0.000582209],[7,3])
      settings: InputPortMap=u0,u1
  ZudX1 q+5 : Lookup_n-D  BreakpointsForDimension1=[-30 -20 -10 0 10 20 30]  BreakpointsForDimension2=[-35.0624 -15.3724 -13.8724]  BreakpointsForDimension3=[-35.0624 -15.3724 -13.8724]  Table=|  InternalRulePriority=Speed  RndMeth=Simplest  InputSameDT=on
      | reshape([-0.000461714
      | -0.000296336
      | -0.000130959
      | 3.44194E-05
      | 0.000199797
      | 0.000365175
      | 0.000530553
      | -0.000503641
      | -0.000327652
      | -0.000151663
      | 2.43257E-05
      | 0.000200315
      | 0.000376303
      | 0.000552292
      | -0.000536558
      | -0.000356664
      | -0.00017677
      | 3.1235E-06
      | 0.000183017
      | 0.000362911
      | 0.000542805],[7,3])
      settings: InputPortMap=u0,u1
  MdX : Outport
  wires:
  Demux6/5 -> ZudX1 q+5/1
  Demux6/4 -> ZudX1 q+4/1
  Demux6/3 -> ZudX1 q+3/1
  Demux6/2 -> ZudX1 q+2/1
  ZudX1 q+4/1 -> Mux/4
  ZudX1 q+3/1 -> Mux/3
  ZudX1 q+2/1 -> Mux/2
  ZudX1 q+1/1 -> Mux/1
  ZudX1 q+5/1 -> Mux/5
  z/1 -> ZudX1 q+5/2, ZudX1 q+4/2, ZudX1 q+3/2, ZudX1 q+2/2, ZudX1 q+1/2
  Mux/1 -> MdX/1
  Demux6/1 -> ZudX1 q+1/1
  dX/1 -> Demux6/1

== system Model_6DOF_B3/HDM B1/N/NdXi ==
  dX : Inport
  z : Inport  Port=2
  Mux : Mux
  NdX1 : Lookup_n-D  BreakpointsForDimension1=[-10 0 10]  BreakpointsForDimension2=|  BreakpointsForDimension3=[-5.14444 -3.08666664 -1.54332]  Table=|  InternalRulePriority=Speed  RndMeth=Simplest  InputSameDT=on
      BreakpointsForDimension2=|
      | [-36.4062987
      | -18.4062987
      | -15.4062987
      | -13.9062987]
      Table=|
      | reshape([-8.13475E-05
      | -3.25752E-06
      | 6.9363E-05
      | -8.00129E-05
      | -1.7093E-06
      | 7.14001E-05
      | -6.46417E-05
      | -1.7093E-06
      | 8.57128E-05
      | -7.85432E-05
      | -1.19372E-08
      | 7.37459E-05],[3,4])
      settings: InputPortMap=u0,u1
  NdX2 : Lookup_n-D  BreakpointsForDimension1=[-10 0 10]  BreakpointsForDimension2=|  BreakpointsForDimension3=[-5.14444 -3.08666664 -1.54332]  Table=|  InternalRulePriority=Speed  RndMeth=Simplest  InputSameDT=on
      BreakpointsForDimension2=|
      | [-36.4062987
      | -18.4062987
      | -15.4062987
      | -13.9062987]
      Table=|
      | reshape([6.2278E-05
      | -3.5277E-06
      | -7.1028E-05
      | 5.9473E-05
      | -6.2352E-06
      | -7.5067E-05
      | 3.9525E-05
      | -6.2352E-06
      | -9.4282E-05
      | 5.5892E-05
      | -1.0640E-05
      | -8.2654E-05],[3,4])
      settings: InputPortMap=u0,u1
  NdX3 : Lookup_n-D  BreakpointsForDimension1=[-10 0 10]  BreakpointsForDimension2=|  BreakpointsForDimension3=[-5.14444 -3.08666664 -1.54332]  Table=|  InternalRulePriority=Speed  RndMeth=Simplest  InputSameDT=on
      BreakpointsForDimension2=|
      | [-36.4062987
      | -18.4062987
      | -15.4062987
      | -13.9062987]
      Table=|
      | reshape([8.96891E-05
      | 3.65995E-06
      | -8.07998E-05
      | 9.13096E-05
      | 6.34009E-06
      | -7.59117E-05
      | 0.000100356
      | 6.34009E-06
      | -4.56822E-05
      | 9.40576E-05
      | 1.06795E-05
      | -6.79415E-05],[3,4])
      settings: InputPortMap=u0,u1
  NdX4 : Lookup_n-D  BreakpointsForDimension1=[-10 0 10]  BreakpointsForDimension2=|  BreakpointsForDimension3=[-5.14444 -3.08666664 -1.54332]  Table=|  InternalRulePriority=Speed  RndMeth=Simplest  InputSameDT=on
      BreakpointsForDimension2=|
      | [-36.4062987
      | -18.4062987
      | -15.4062987
      | -13.9062987]
      Table=|
      | reshape([-7.16232E-05
      | 3.25314E-06
      | 8.32589E-05
      | -7.3213E-05
      | 1.68586E-06
      | 8.13825E-05
      | -8.66615E-05
      | 1.68586E-06
      | 6.54218E-05
      | -7.48528E-05
      | -6.7812E-08
      | 7.92559E-05],[3,4])
      settings: InputPortMap=u0,u1
  Selector1 : Selector  InputPortWidth=5  IndexOptions=Index vector (dialog)  Indices=2  OutputSizes=1
  Selector2 : Selector  InputPortWidth=5  IndexOptions=Index vector (dialog)  Indices=3  OutputSizes=1
  Selector3 : Selector  InputPortWidth=5  IndexOptions=Index vector (dialog)  Indices=4  OutputSizes=1
  Selector7 : Selector  InputPortWidth=5  IndexOptions=Index vector (dialog)  Indices=1  OutputSizes=1
  NdXi : Outport
  wires:
  Selector3/1 -> NdX4/1
  Selector2/1 -> NdX3/1
  Selector1/1 -> NdX2/1
  NdX4/1 -> Mux/4
  NdX3/1 -> Mux/3
  NdX2/1 -> Mux/2
  NdX1/1 -> Mux/1
  z/1 -> NdX1/2, NdX2/2, NdX3/2, NdX4/2
  Mux/1 -> NdXi/1
  Selector7/1 -> NdX1/1
  dX/1 -> Selector7/1, Selector1/1, Selector2/1, Selector3/1

== system Model_6DOF_B3/HDM B1/Wave, Virtual Mass and Hydrostatic/Wave Particle Motions ==
  U_ship : Inport
  X_earth : Inport  Port=2
  CGi : Inport  Port=3
  CG : Inport  Port=4
  SeaState : Inport  Port=5
  dLCG : Inport  Port=6
  Add : Sum  Inputs=+-
  Clock : Clock
  Constant : Constant  Value=3
  Constant1 : Constant  Value=Zb
  Constant2 : Constant  Value=0.4406
  Constant6 : Constant  Value=1025
  Constant7 : Constant  Value=9.81
  Derivative : Derivative
  Derivative1 : Derivative
  Local eff. Depth : MATLAB Function  TreatAsAtomicUnit=on
  MATLAB Function1 : MATLAB Function  TreatAsAtomicUnit=on
  Mux : Mux  Inputs=5
  Sectional Position Vectors : MATLAB Function  TreatAsAtomicUnit=on
  Sectional Wave Particle & Rigid Body Velocities : MATLAB Function  TreatAsAtomicUnit=on
  Subsystem : Subsystem
  Wave Properties : MATLAB Function  TreatAsAtomicUnit=on
  Wave particle velocity at hull CG : MATLAB Function  TreatAsAtomicUnit=on
  X_SP1 : Constant  Value=[31.924; 3.861; -3.861;]
  X_SP2 : Constant  Value=[31.924; 3.861; 3.861;]
  X_SP3 : Constant  Value=[31.924; -3.861; 3.861;]
  X_SP4 : Constant  Value=[31.924; -3.861; -3.861;]
  X_XB : Constant  Value=[-10.465; 0; 9.732;]
  beta_wave : Constant  Value=0
  phi_wave : Constant  Value=0
  aws : Outport
  ars : Outport  Port=2
  Rs : Outport  Port=3
  zeff : Outport  Port=4
  uwXis : Outport  Port=5
  uwsCG : Outport  Port=6
  uws : Outport  Port=7
  urs : Outport  Port=8
  B_FM : Outport  Port=9
  wires:
  Constant1/1 -> Add/2
  Constant2/1 -> Add/1
  Add/1 -> Subsystem/8(Zb)
  Constant7/1 -> Subsystem/7(g)
  Constant6/1 -> Subsystem/6(rho)
  Subsystem/1(Out1) -> B_FM/1
  Constant/1 -> Sectional Wave Particle & Rigid Body Velocities/12(iProbe)
  Wave particle velocity at hull CG/1(uwsCG) -> uwsCG/1
  beta_wave/1 -> Wave particle velocity at hull CG/6(beta_wave), Sectional Wave Particle & Rigid Body Velocities/7(beta_wave), MATLAB Function1/11(beta_wave)
  phi_wave/1 -> MATLAB Function1/10(phi_wave), Wave particle velocity at hull CG/5(phi_wave), Sectional Wave Particle & Rigid Body Velocities/6(phi_wave)
  Mux/1 -> uwXis/1
  MATLAB Function1/5(uwXBs) -> Mux/5
  MATLAB Function1/4(uwX4s) -> Mux/4
  MATLAB Function1/3(uwX3s) -> Mux/3
  MATLAB Function1/2(uwX2s) -> Mux/2
  MATLAB Function1/1(uwX1s) -> Mux/1
  X_SP1/1 -> MATLAB Function1/2(rX1)
  X_SP2/1 -> MATLAB Function1/3(rX2)
  X_SP3/1 -> MATLAB Function1/4(rX3)
  X_SP4/1 -> MATLAB Function1/5(rX4)
  X_XB/1 -> MATLAB Function1/6(rXB)
  Local eff. Depth/1(z_eff) -> zeff/1
  Wave Properties/2(A_wave) -> Sectional Wave Particle & Rigid Body Velocities/9(A_wave), MATLAB Function1/12(A_wave), Local eff. Depth/5(a_wave), Wave particle velocity at hull CG/7(A_wave), Subsystem/3(A_wave)
  dLCG/1 -> Sectional Position Vectors/4(dLCG), Wave particle velocity at hull CG/3(dLCG)
  Derivative1/1 -> ars/1
  Sectional Wave Particle & Rigid Body Velocities/1(Uws) -> uws/1, Derivative/1
  Sectional Wave Particle & Rigid Body Velocities/2(Urs) -> urs/1, Derivative1/1
  CG/1 -> Sectional Position Vectors/3(CG)
  CGi/1 -> Sectional Position Vectors/2(CGi)
  Derivative/1 -> aws/1
  Wave Properties/4(w_wave) -> Sectional Wave Particle & Rigid Body Velocities/11(w_wave), MATLAB Function1/14(w_wave), Local eff. Depth/4(w_wave), Wave particle velocity at hull CG/9(w_wave), Subsystem/5(w_wave)  "w"
  Wave Properties/1(L_wave) -> Wave particle velocity at hull CG/4(L_wave), Sectional Wave Particle & Rigid Body Velocities/8(L_wave), MATLAB Function1/9(L_wave)
  U_ship/1 -> Sectional Wave Particle & Rigid Body Velocities/2(U_ship), MATLAB Function1/8(U_ship)
  Wave Properties/3(k_wave) -> Sectional Wave Particle & Rigid Body Velocities/10(k_wave), MATLAB Function1/13(k_wave), Local eff. Depth/3(k_wave), Wave particle velocity at hull CG/8(k_wave), Subsystem/4(k_wave)  "k"
  X_earth/1 -> Sectional Position Vectors/1(X_earth), Local eff. Depth/2(Bxe), Wave particle velocity at hull CG/2(X_earth), MATLAB Function1/7(X_earth), Sectional Wave Particle & Rigid Body Velocities/3(X_earth), Subsystem/2(Xearth)
  Sectional Position Vectors/1(Xce) -> Sectional Wave Particle & Rigid Body Velocities/4(Xce)
  Clock/1 -> Sectional Wave Particle & Rigid Body Velocities/1(time), Local eff. Depth/1(time), Wave particle velocity at hull CG/1(time), MATLAB Function1/1(time), Subsystem/1(time)
  SeaState/1 -> Wave Properties/1(SeaState)
  Sectional Position Vectors/2(Rs) -> Rs/1, Sectional Wave Particle & Rigid Body Velocities/5(Rs)
